simulink model "LAB_01_19_SEPT_SIM_ES"  (R2022b)
settings: Solver=VariableStepAuto  StartTime=0.0  StopTime=10.0  RelTol=1e-3
values from neighbouring files (symbols this model uses):
  g = 9.81    [LAB_02_26_SEPT_MAT_PENDULUM.m]
  l = strcat([h,'',i])    [LAB_01_19_SEPT.m]    (also in LAB_02_26_SEPT_MAT_PENDULUM.m = 5)
undefined symbols (not defined in the file or in its folder): w_0
settings Model: Creator=maria  LastModifiedBy=maria

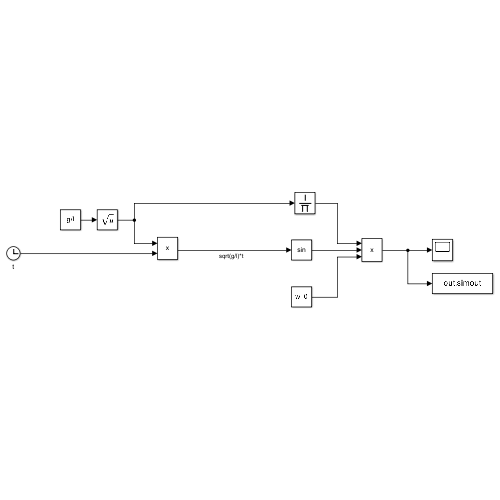
[thumbnail: Simulink's stored preview of the top-level diagram]
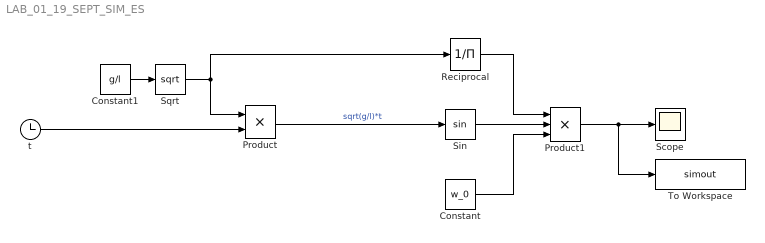
== system LAB_01_19_SEPT_SIM_ES ==
  Constant : Constant  Value=w_0
  Constant1 : Constant  Value=g/l
  Product : Product
  Product1 : Product  Inputs=3
  Reciprocal : Product  Inputs=/  RndMeth=Zero  SaturateOnIntegerOverflow=on
  Scope : Scope
  Sin : Trigonometry
  Sqrt : Sqrt
  To Workspace : ToWorkspace  VariableName=simout  SaveFormat=Timeseries  SampleTime=-1
  t : Clock
  wires:
  Constant1/1 -> Sqrt/1
  Sqrt/1 -> Reciprocal/1, Product/1
  t/1 -> Product/2
  Product/1 -> Sin/1  "sqrt(g/l)*t"
  Sin/1 -> Product1/2
  Reciprocal/1 -> Product1/1
  Constant/1 -> Product1/3
  Product1/1 -> To Workspace/1, Scope/1
